simulink model "ej3"  (Simulink 8.5)
settings: Solver=ode45  StartTime=0.0  StopTime=3  RelTol=1e-3
settings Model: Creator=alumno  LastModifiedBy=dani
settings DataIOCC: LimitDataPoints=off
settings OptimizationCC: InitFltsAndDblsToZero=on
settings DebuggingCC: SolverPrmCheckMsg=warning  FcnCallInpInsideContextMsg=UseLocalSettings

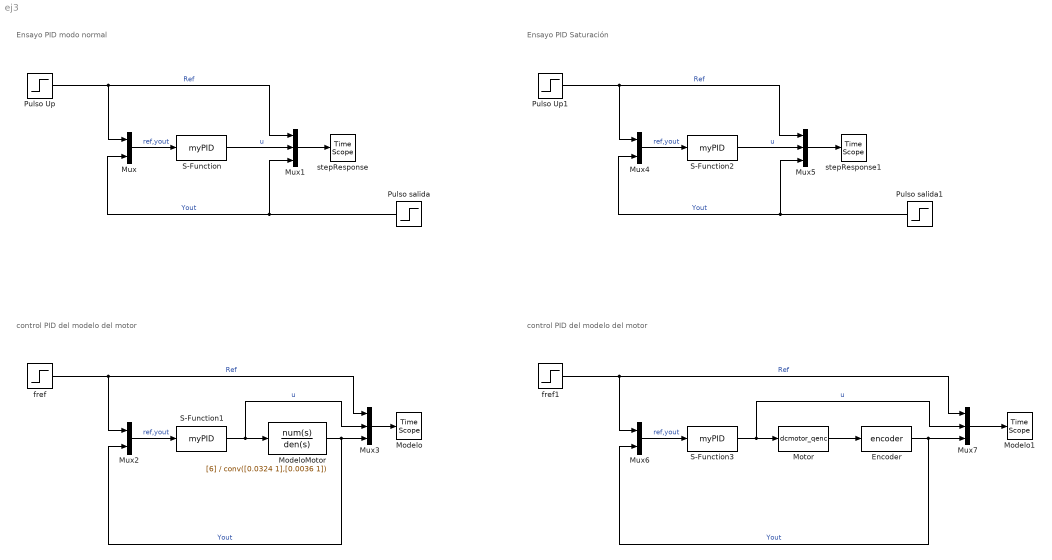
== system ej3 ==
  note: Ensayo PID modo normal
  note: control PID del modelo del motor
  note: Ensayo PID Saturación
  note: control PID del modelo del motor
  Encoder : S-Function  FunctionName=encoder  Parameters=1E-5 10
  Modelo : TimeScope
  Modelo1 : TimeScope
  ModeloMotor : TransferFcn  Numerator=[6]  Denominator=conv([0.0324 1],[0.0036 1])
  Motor : S-Function  FunctionName=dcmotor_qenc  Parameters=10
  Mux{,2,4,6} (4 alike) : Mux  Inputs=2
  Mux{1,3,5,7} (4 alike) : Mux  Inputs=3
  Pulso Up : Step  SampleTime=0
  Pulso Up1 : Step  SampleTime=0
  Pulso salida : Step  Time=2  SampleTime=0
  Pulso salida1 : Step  Time=2  SampleTime=0
  S-Function : S-Function  FunctionName=myPID  Parameters=1 0.1 1 1 1E-3
  S-Function1 : S-Function  FunctionName=myPID  Parameters=1 0.01 10 10 1E-3 0 24
  S-Function2 : S-Function  FunctionName=myPID  Parameters=1 0.1 1 1 1E-3 -10 1.5
  S-Function3 : S-Function  FunctionName=myPID  Parameters=1 0.01 10 10 1E-3 0 24
  fref : Step  After=45  SampleTime=0
  fref1 : Step  After=45  SampleTime=0
  stepResponse : TimeScope
  stepResponse1 : TimeScope
  wires:
  Pulso Up/1 -> Mux1/1, Mux/1  "Ref"
  Mux1/1 -> stepResponse/1
  S-Function/1 -> Mux1/2  "u"
  Mux/1 -> S-Function/1  "ref,yout"
  Pulso salida/1 -> Mux/2, Mux1/3  "Yout"
  fref/1 -> Mux3/1, Mux2/1  "Ref"
  Mux3/1 -> Modelo/1
  S-Function1/1 -> Mux3/2, ModeloMotor/1  "u"
  Mux2/1 -> S-Function1/1  "ref,yout"
  ModeloMotor/1 -> Mux3/3, Mux2/2  "Yout"
  Pulso Up1/1 -> Mux5/1, Mux4/1  "Ref"
  Mux5/1 -> stepResponse1/1
  S-Function2/1 -> Mux5/2  "u"
  Mux4/1 -> S-Function2/1  "ref,yout"
  Pulso salida1/1 -> Mux4/2, Mux5/3  "Yout"
  fref1/1 -> Mux7/1, Mux6/1  "Ref"
  Mux7/1 -> Modelo1/1
  S-Function3/1 -> Mux7/2, Motor/1  "u"
  Mux6/1 -> S-Function3/1  "ref,yout"
  Motor/1 -> Encoder/1
  Encoder/1 -> Mux7/3, Mux6/2  "Yout"
